simulink model "module"  (R2015b)
settings: Solver=ode45  StartTime=0.0  StopTime=10.0  RelTol=1e-3
undefined symbols (not defined in the file): Ts
libraries: commrandsrc3 x1
settings Model: Creator=leejitang  LastModifiedBy=votex
settings DataIOCC: SaveFormat=Array  SignalLoggingSaveFormat=ModelDataLogs
settings OptimizationCC: ExpressionDepthLimit=2147483647
settings DebuggingCC: UnderspecifiedInitializationDetection=Classic  MergeDetectMultiDrivingBlocksExec=none  SolverPrmCheckMsg=warning  FcnCallInpInsideContextMsg=EnableAllAsWarning  StateNameClashWarn=warning
settings HardwareCC: ProdBitPerPointer=32  ProdLargestAtomicFloat=None  ProdIntDivRoundTo=Undefined  ProdEndianess=Unspecified  ProdWordSize=32  ProdHWDeviceType=32-bit Generic
settings GRTTargetCC: GeneratePreprocessorConditionals=Disable all
settings ConfigComp: CovModelRefEnable=Off

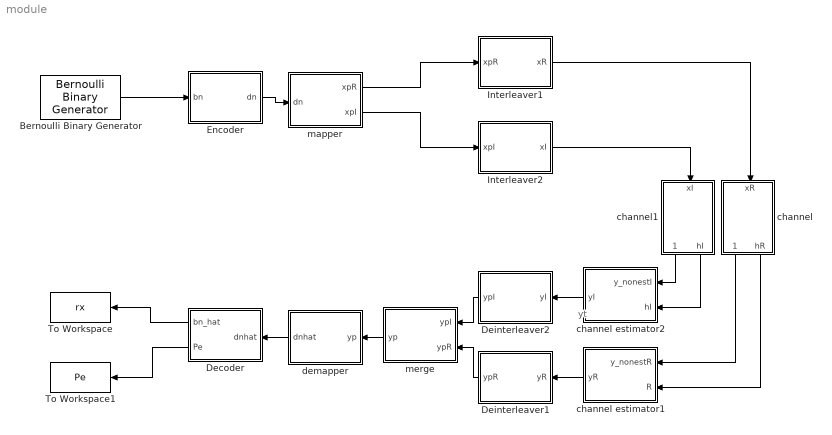
== system module ==
  note: yt
  Bernoulli Binary Generator : commrandsrc3/Bernoulli Binary Generator  ProbabilityOfZero=0.5  SeedSource=Auto  Seed=0  SampleTime=Ts  SamplesPerFrame=2  OutputDataType=double  SimulateUsing=Interpreted execution
  Decoder : MATLAB Function  TreatAsAtomicUnit=on
  Deinterleaver1 : MATLAB Function  TreatAsAtomicUnit=on
  Deinterleaver2 : MATLAB Function  TreatAsAtomicUnit=on
  Encoder : MATLAB Function  TreatAsAtomicUnit=on
  Interleaver1 : MATLAB Function  TreatAsAtomicUnit=on
  Interleaver2 : MATLAB Function  TreatAsAtomicUnit=on
  To Workspace : ToWorkspace  VariableName=rx  SampleTime=-1
  To Workspace1 : ToWorkspace  VariableName=Pe  SampleTime=-1
  channel : MATLAB Function  TreatAsAtomicUnit=on
  channel estimator1 : MATLAB Function  TreatAsAtomicUnit=on
  channel estimator2 : MATLAB Function  TreatAsAtomicUnit=on
  channel1 : MATLAB Function  TreatAsAtomicUnit=on
  demapper : MATLAB Function  TreatAsAtomicUnit=on
  mapper : MATLAB Function  TreatAsAtomicUnit=on
  merge : MATLAB Function  TreatAsAtomicUnit=on
  wires:
  Bernoulli Binary Generator/1 -> Encoder/1(bn)
  Decoder/1(bn_hat) -> To Workspace/1
  channel/1(y_nonestI) -> channel estimator1/1(y_nonestR)
  channel/2(hR) -> channel estimator1/2(R)
  Decoder/2(Pe) -> To Workspace1/1
  Deinterleaver2/1(ypI) -> merge/1(ypI)
  Deinterleaver1/1(ypR) -> merge/2(ypR)
  Interleaver2/1(xI) -> channel1/1(xI)
  Interleaver1/1(xR) -> channel/1(xR)
  channel estimator2/1(yI) -> Deinterleaver2/1(yI)
  channel estimator1/1(yR) -> Deinterleaver1/1(yR)
  channel1/1(y_nonestI) -> channel estimator2/1(y_nonestI)
  channel1/2(hI) -> channel estimator2/2(hI)
  Encoder/1(dn) -> mapper/1(dn)
  merge/1(yp) -> demapper/1(yp)
  mapper/1(xpR) -> Interleaver1/1(xpR)
  mapper/2(xpI) -> Interleaver2/1(xpI)
  demapper/1(dnhat) -> Decoder/1(dnhat)

== matlab function module/Encoder ==
  data: bn input; dn output
function dn = f(bn)

% repetition code
% codeword length n = 3
% information bit k = 1
n = 2;
k = 1;

[I, J] = size(b);
d = zeros(6,J*n);
m = eye(2);
end

== matlab function module/Decoder ==
  data: dnhat input; bn_hat output; Pe output
function [bn_hat,Pe] = f(dnhat)

bn_hat = b(:,1);


end

== matlab function module/Interleaver2 ==
  data: xpI input; xI output
function xI = in(xpI)

dn = dn(1:2)';

s = 1/sqrt(2);
if isequal(dn,[1,1])
    x = s;
    y = s;

elseif isequal(dn,[0,1])
    x = -s;
    y = s;

elseif isequal(dn,[1,0])
    x = s;
    y = -s;

else
    x = -s;
    y = -s;
end
d = x+1j*y;
end

== matlab function module/Deinterleaver2 ==
  data: yI input; ypI output
function ypI = de_in(yI)

yp = yp(1:2)';

s = 1/sqrt(2);
if isequal(yp,[1,1])
    x = s;
    y = s;

elseif isequal(yp,[0,1])
    x = -s;
    y = s;

elseif isequal(yp,[1,0])
    x = s;
    y = -s;

else
    x = -s;
    y = -s;
end
b = x+1j*y;
end

== matlab function module/channel estimator1 ==
  data: y_nonestR input; yR output; R input
function yR = d(y_nonestR, R)


z = y';
a = real(z);
b = imag(z);
pos = [a,b];

bithat = [a>0 b>0];

bithat = double(bithat);

yt = bithat(:);

end

== matlab function module/mapper ==
  data: xpR output; dn input; xpI output
function [xpR,xpI] = map(dn)

dn = dn(1:2)';

s = 1/sqrt(2);
if isequal(dn,[1,1])
    x1 = s;
    y1 = s;

elseif isequal(dn,[0,1])
    x1 = -s;
    y1 = s;

elseif isequal(dn,[1,0])
    x1 = s;
    y1 = -s;

else
    x1 = -s;
    y1 = -s;
end
x = x1+1j*y1;
end

== matlab function module/channel ==
  data: xR input; y_nonestI output; hR output
function [y_nonestI, hR] = Rayleigh(xR)

% y[m] = h_0[m]*x[m] + w[m]
sigma_h = 1;
sigma_w = 5; % set in main file??
N = size(x,1);
r = sigma_h.*(randn(N,1));
w = sigma_w.*(randn(N,1));
h = r.*exp(1j*2*pi*rand(N,1)) + w;
y = h.*x;
% y = 0;
end

== matlab function module/demapper ==
  data: yp input; dnhat output
function dnhat = d(yp)


z = yt';
a = real(z);
b = imag(z);
pos = [a,b];

bithat = [a>0 b>0];

bithat = double(bithat);

yp = bithat(:);

end

== matlab function module/Interleaver1 ==
  data: xpR input; xR output
function xR = in(xpR)

dn = dn(1:2)';

s = 1/sqrt(2);
if isequal(dn,[1,1])
    x = s;
    y = s;

elseif isequal(dn,[0,1])
    x = -s;
    y = s;

elseif isequal(dn,[1,0])
    x = s;
    y = -s;

else
    x = -s;
    y = -s;
end
d = x+1j*y;
end

== matlab function module/Deinterleaver1 ==
  data: yR input; ypR output
function ypR = de_in(yR)

yp = yp(1:2)';

s = 1/sqrt(2);
if isequal(yp,[1,1])
    x = s;
    y = s;

elseif isequal(yp,[0,1])
    x = -s;
    y = s;

elseif isequal(yp,[1,0])
    x = s;
    y = -s;

else
    x = -s;
    y = -s;
end
b = x+1j*y;
end

== matlab function module/merge ==
  data: ypI input; yp output; ypR input
function yp = d(ypI, ypR)


z = yt';
a = real(z);
b = imag(z);
pos = [a,b];

bithat = [a>0 b>0];

bithat = double(bithat);

yp = bithat(:);

end

== matlab function module/channel1 ==
  data: xI input; y_nonestI output; hI output
function [y_nonestI, hI] = Rayleigh(xI)

% y[m] = h_0[m]*x[m] + w[m]
sigma_h = 1;
sigma_w = 5; % set in main file??
N = size(x,1);
r = sigma_h.*(randn(N,1));
w = sigma_w.*(randn(N,1));
h = r.*exp(1j*2*pi*rand(N,1)) + w;
y = h.*x;
% y = 0;
end

== matlab function module/channel estimator2 ==
  data: y_nonestI input; yI output; hI input
function yI = d(y_nonestI, hI)


z = y';
a = real(z);
b = imag(z);
pos = [a,b];

bithat = [a>0 b>0];

bithat = double(bithat);

yt = bithat(:);

end
